simulink model "PV_MG_DroopMPPTVx_OneFarm"  (Simulink 8.5)
settings: Solver=ode3  StartTime=0.0  StopTime=inf  FixedStep=DT  RelTol=1e-3
PreLoadFcn:
  | DTCTinit;
PostLoadFcn:
  | Ts=50e-6;
InitFcn:
  | DTCTinit;
undefined symbols (not defined in the file): CT, DT
libraries: powerlib x25, simulink x6, powerlib_meascontrol x4, rtlab x2, simulink_extras x1, re_lib x1
settings Model: Creator=Nady  LastModifiedBy=ga63vey  PauseTimes=1.45  CovModelRefEnable=off
settings DataIOCC: SaveFormat=StructureWithTime  SignalLoggingSaveFormat=Dataset
settings OptimizationCC: ExpressionDepthLimit=128
settings DebuggingCC: UnderspecifiedInitializationDetection=Simplified  MergeDetectMultiDrivingBlocksExec=error  FcnCallInpInsideContextMsg=EnableAllAsError  StateNameClashWarn=none
settings HardwareCC: ProdBitPerPointer=64  ProdLargestAtomicFloat=Float  ProdIntDivRoundTo=Zero  ProdEndianess=LittleEndian  ProdHWDeviceType=Specified
settings GRTTargetCC: GeneratePreprocessorConditionals=Use local settings  CombineOutputUpdateFcns=on  GRTInterface=off

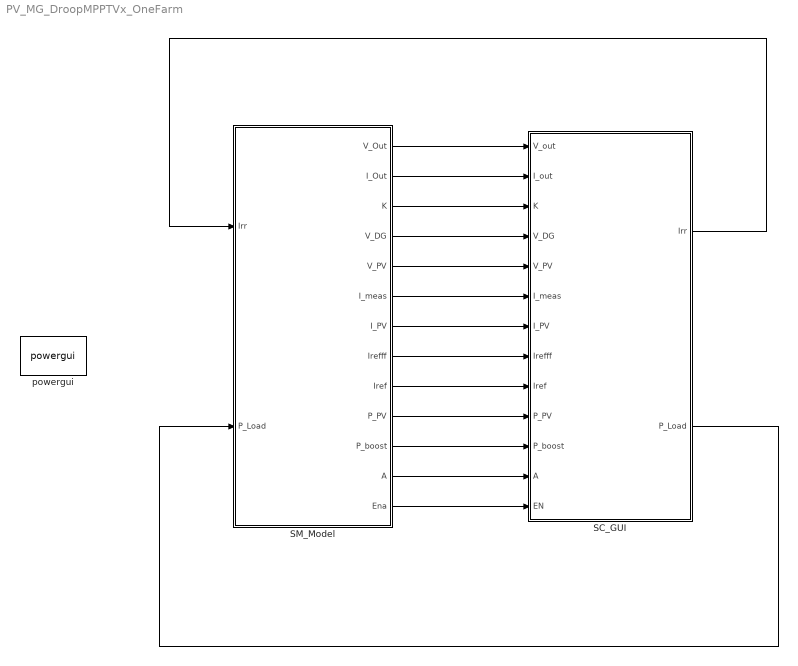
== system PV_MG_DroopMPPTVx_OneFarm ==
  SC_GUI : Subsystem
  SM_Model : Subsystem
  powergui : powerlib/powergui  Priority=1  SimulationMode=Discrete  SolverType=Tustin  SampleTime=DT  frequency=60  SPID=off  DisableSnubberDevices=off  DisableRonSwitches=off  DisableVfSwitches=off  SwTol=0  DisplayEquations=off  Interpol=off  methode=on  Ts=20  FunctionMessages=off  echomessages=off  HookPort=off  EnableUseOfTLC=off  x0status=blocks  frequencyindice=0  Pbase=100e6  ErrMax=1e-4  Iterations=50  UnitsV=kV  UnitsW=MW  buscounter=0  RestoreLinks=warning  ResistiveCurrentMeasurement=off  Frange=[0:2:500]  Ylog=off  Xlog=on  ShowGrid=off  save=off  variable=ZData  structure=0  ZoomFFT=off  StartTime=0.0  cycles=1  DisplayStyle=1  fundamental=60  FreqAxis=off  MaxFrequency=1000  frequencyindicesteady=1  RmsSteady=1  display=off
  wires:
  SC_GUI/1(Irr) -> SM_Model/1(Irr)
  SC_GUI/2(P_Load) -> SM_Model/2(P_Load)
  SM_Model/1(V_Out) -> SC_GUI/1(V_out)
  SM_Model/2(I_Out) -> SC_GUI/2(I_out)
  SM_Model/3(K) -> SC_GUI/3(K)
  SM_Model/4(V_DG) -> SC_GUI/4(V_DG)
  SM_Model/5(V_PV) -> SC_GUI/5(V_PV)
  SM_Model/6(I_meas) -> SC_GUI/6(I_meas)
  SM_Model/7(I_PV) -> SC_GUI/7(I_PV)
  SM_Model/8(Irefff) -> SC_GUI/8(Irefff)
  SM_Model/9(Iref) -> SC_GUI/9(Iref)
  SM_Model/10(P_PV) -> SC_GUI/10(P_PV)
  SM_Model/11(P_boost) -> SC_GUI/11(P_boost)
  SM_Model/12(A) -> SC_GUI/12(A)
  SM_Model/13(Ena) -> SC_GUI/13(EN)

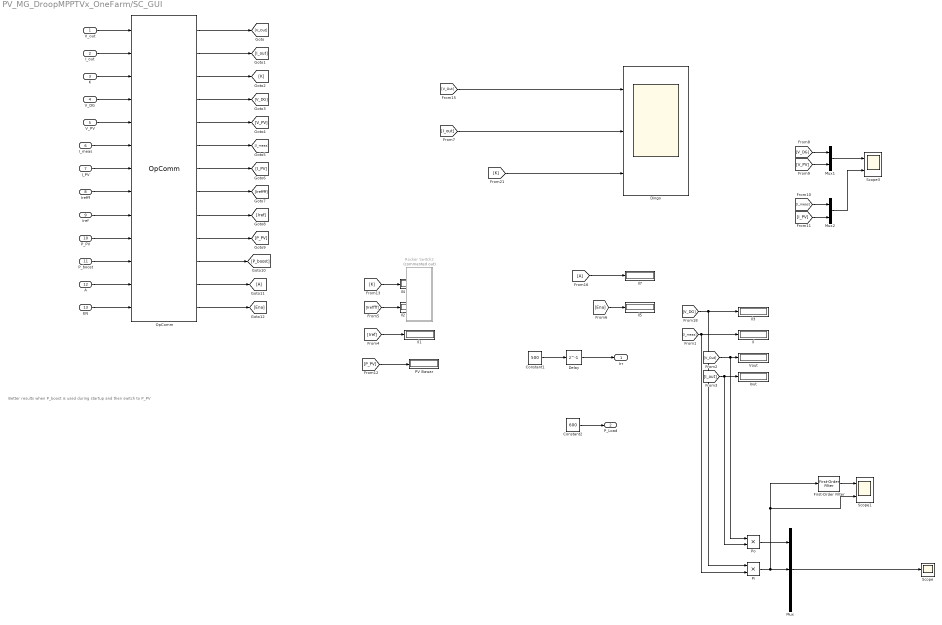
== system PV_MG_DroopMPPTVx_OneFarm/SC_GUI ==
  note: Better results when P_boost is used during startup and then switch to P_PV
  V_out : Inport
  I_out : Inport  Port=2
  K : Inport  Port=3
  V_DG : Inport  Port=4
  V_PV : Inport  Port=5
  I_meas : Inport  Port=6
  I_PV : Inport  Port=7
  Irefff : Inport  Port=8
  Iref : Inport  Port=9
  P_PV : Inport  Port=10
  P_boost : Inport  Port=11
  A : Inport  Port=12
  EN : Inport  Port=13
  Constant1 : Constant  Value=500  SampleTime=0
  Constant2 : Constant  Value=600  SampleTime=0
  Delay : Delay  DelayLength=1  InitialCondition=0
  Dingo : Scope  NumInputPorts=3
      settings: ShowLegends=on  TimeRange=3.8087  YMin=0~0~0  YMax=400~1.2~1.4  MaxDataPoints=10000
  First-Order Filter : powerlib_meascontrol/Filters/First-Order Filter  FilterType=Lowpass  Tc=1/400  Ts=DT  Initialize=off  Vac_Init=[0, 0, 60]  Vdc_Init=0  PlotResponse=off  FreqRange="[0,  200,  1]"
  Il{,1..5,7} (7 alike) : Display
  Iout : Display
  Mux : Mux  Inputs=3
  Mux1 : Mux  Inputs=2
  Mux2 : Mux  Inputs=2
  OpComm : rtlab/OpComm  nbport=13  groupe_acq=1  subsys_rate=0  st=0  Synchronization=on  Interpolation=on  Threshold=1.0  Missed_Data=off  Sim_Time=off  Samples=off  dynSigOut=off  from_console=0  warning_done=off  writeOpCommFile=off  Offset=off
  PV Bawar : Display
  Pi : Product
  Po : Product
  Rocker Switch2 : Subsystem  Commented=on  DialogController=hmiCreateDDGDialog  DialogControllerArgs=DataTag0  mask(MWDashboardBlock){webBlockId=5e99b1b3-df07-4cef-a3f6-0ddfeeb3b4e9, webBlockType=rockerswitch, ShowInLibBrowser=on, ShowInitialText=on, HMISrcModelName=[]}
      mask prompts: webBlockId "WebBlock Id"; webBlockType "WebBlock Type"; HMISrcModelName "Source Model"
      mask Help: helpview([docroot '/mapfiles/simulink.map'], 'hmi_rocker_switch')
      mask Display:
      | if strcmp(get_param(bdroot(gcb),'BlockDiagramType'), 'library')
      |     image([(matlabroot) '/toolbox/simulink/hmi/icons/RockerSwitch.png']);
      | end
  Scope : Scope
      settings: ShowLegends=on  YMin=-107.077  YMax=623.287  MaxDataPoints=10000
  Scope1 : Scope  NumInputPorts=2
      settings: YMin=-102.309~-5  YMax=495.80827~5
  Scope3 : Scope  NumInputPorts=2
      settings: YMin=-2.6975~-3.12322  YMax=24.27751~28.10897  SaveName=ScopeData3
  Vout : Display
  Irr : Outport
  P_Load : Outport  Port=2
  wires:
  [I_meas] -> Pi/2, Il/1
  [V_Out] -> Po/1, Vout/1
  [I_out] -> Po/2, Iout/1
  [V_DG] -> Il3/1, Pi/1
  Po/1 -> Mux/1
  Pi/1 -> First-Order Filter/1, Scope1/2, Mux/2
  [Iref] -> Il1/1
  [Ireffff] -> Il2/1
  [Ena] -> Il5/1
  First-Order Filter/1 -> Scope1/1
  Mux1/1 -> Scope3/1
  [V_DG] -> Mux1/1
  [V_PV] -> Mux1/2
  Mux2/1 -> Scope3/2
  [I_meas] -> Mux2/1
  [I_PV] -> Mux2/2
  [P_PV] -> PV Bawar/1
  [K] -> Il4/1
  Mux/1 -> Scope/1
  [K] -> Dingo/3
  [V_Out] -> Dingo/1
  [I_out] -> Dingo/2
  Constant1/1 -> Delay/1
  [A] -> Il7/1
  Delay/1 -> Irr/1
  V_out/1 -> OpComm/1
  I_out/1 -> OpComm/2
  K/1 -> OpComm/3
  V_DG/1 -> OpComm/4
  V_PV/1 -> OpComm/5
  I_meas/1 -> OpComm/6
  I_PV/1 -> OpComm/7
  Irefff/1 -> OpComm/8
  Iref/1 -> OpComm/9
  P_PV/1 -> OpComm/10
  P_boost/1 -> OpComm/11
  OpComm/1 -> [V_Out]
  OpComm/2 -> [I_out]
  OpComm/3 -> [K]
  OpComm/4 -> [V_DG]
  OpComm/5 -> [V_PV]
  OpComm/6 -> [I_meas]
  OpComm/7 -> [I_PV]
  OpComm/8 -> [Ireffff]
  OpComm/9 -> [Iref]
  OpComm/10 -> [P_PV]
  OpComm/11 -> [P_boost]
  OpComm/12 -> [A]
  OpComm/13 -> [Ena]
  A/1 -> OpComm/12
  EN/1 -> OpComm/13
  Constant2/1 -> P_Load/1

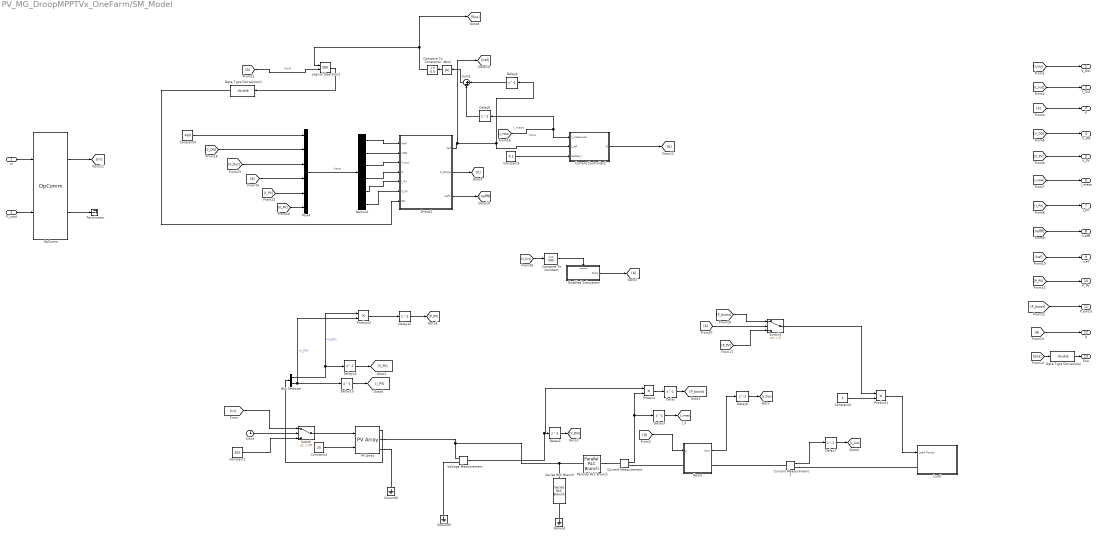
== system PV_MG_DroopMPPTVx_OneFarm/SM_Model ==
  note: here
  note: here
  note: here
  note: I_meas
  Irr : Inport
  P_Load : Inport  Port=2
  Abs2 : Abs
  Boost : Subsystem
  Bus Selector : BusSelector  OutputSignals=V_PV,I_PV
  Clock : Clock
  Compare To Constant : simulink/Logic and Bit Operations/Compare To Constant  relop=>=  const=395  OutDataTypeStr=boolean
  Compare To Constant2 : simulink/Logic and Bit Operations/Compare To Constant  relop=<=  const=0.5  OutDataTypeStr=boolean
  Constant1 : Constant  Value=400  SampleTime=0
  Constant2 : Constant  Value=25
  Constant3 : Constant  SampleTime=0
  Constant4 : Constant  Value=400  SampleTime=DT
  Constant5 : Constant  Value=0.1  SampleTime=CT
  Current Controller2 : Subsystem  TreatAsAtomicUnit=on
  Current Measurement : powerlib/Measurements/Current Measurement  PhasorSimulation=off  OutputType=Complex  PSBequivalent=0
  Current Measurement1 : powerlib/Measurements/Current Measurement  PhasorSimulation=off  OutputType=Complex  PSBequivalent=0
  Data Type Conversion : DataTypeConversion  OutDataTypeStr=double
  Data Type Conversion1 : DataTypeConversion  OutDataTypeStr=double
  Delay{,2..7,12..14} (10 alike) : Delay  DelayLength=1  InitialCondition=0
  Demux1 : Demux  Outputs=6
  Droop2 : Subsystem  TreatAsAtomicUnit=on
  Enabled Subsystem : Subsystem  TreatAsAtomicUnit=on
  Ground : powerlib/Elements/Ground  LConnTagsString=a
  Ground2 : powerlib/Elements/Ground  LConnTagsString=a
  Ground3 : powerlib/Elements/Ground  LConnTagsString=a
  Load : Subsystem
  Logical Operator2 : Logic  Operator=OR  AllPortsSameDT=off  OutDataTypeStr=boolean
  Mux4 : Mux  Inputs=6
  OpComm : rtlab/OpComm  nbport=2  groupe_acq=1  subsys_rate=0  st=0  Synchronization=on  Interpolation=on  Threshold=1.0  Missed_Data=off  Sim_Time=off  Samples=off  dynSigOut=off  from_console=1  warning_done=off  writeOpCommFile=off  Offset=off
  PV Array : re_lib/Solar/PV Array  Npar=5  Nser=1  PlotType=one module @ 25 deg.C & specified irradiances  S_vec="[ 1000  800 ]"  Temp_C_vec=[35]  ModuleName=Sun Earth Solar Power TDB125x125-36-P 80W  PlotWhenSelected=off  Pm=80.004  Ncell=36  Voc=21.9  Isc=5  Vm=17.7  Im=4.52  beta_Voc_pc=-0.32  alpha_Isc_pc=0.04  beta_Voc=-0.07008  alpha_Isc=0.002  IL=5.0238  I0=3.6974e-11  nI=0.92596  Rsh=70.2892  Rs=0.35567  BAL=on  Tc=1e-6  Tfilter=5e-5
  Parallel RLC Branch : powerlib/Elements/Parallel RLC Branch  LConnTagsString=a  RConnTagsString=__new0  BranchType=RL  Resistance=10  Inductance=0.0164  SetiL0=off  InitialCurrent=0  Capacitance=1e-6  Setx0=off  InitialVoltage=0  Measurements=None
  Product : Product
  Product1 : Product
  Product2 : Product
  Series RLC Branch : powerlib/Elements/Series RLC Branch  LConnTagsString=__new0  RConnTagsString=__new0  BranchType=C  Resistance=0.1  Inductance=1e-3  SetiL0=off  InitialCurrent=0  Capacitance=0.1  Setx0=off  InitialVoltage=0  Measurements=None
  Sum2 : Sum  Inputs=|+-
  Switch : Switch  Criteria=u2 > Threshold  Threshold=DT
  Switch1 : Switch  Criteria=u2 > Threshold
  Terminator : Terminator
  Voltage Measurement : powerlib/Measurements/Voltage Measurement  PhasorSimulation=off  OutputType=Complex  PSBequivalent=0
  V_Out : Outport
  I_Out : Outport  Port=2
  K : Outport  Port=3
  V_DG : Outport  Port=4
  V_PV : Outport  Port=5
  I_meas : Outport  Port=6
  I_PV : Outport  Port=7
  Irefff : Outport  Port=8
  Iref : Outport  Port=9
  P_PV : Outport  Port=10
  P_boost : Outport  Port=11
  A : Outport  Port=12
  Ena : Outport  Port=13
  wires:
  Droop2/1(Iref) -> [Iref], Delay4/1, Current Controller2/2(I_ref)
  Constant5/1 -> Current Controller2/3(delata_I)
  Droop2/2(K_droop) -> [K]
  Droop2/3(Iref1) -> [Ireffff]
  Sum2/1 -> Abs2/1
  Abs2/1 -> Compare To Constant2/1
  Delay4/1 -> Sum2/1
  Delay5/1 -> Sum2/2
  Constant4/1 -> Mux4/1
  [V_DG] -> Mux4/2
  [V_Out] -> Mux4/3
  Current Controller2/1(G) -> [G]
  Compare To Constant2/1 -> [Ena], Logical Operator2/1
  Logical Operator2/1 -> Data Type Conversion1/1
  Data Type Conversion1/1 -> Droop2/7(EN)
  Demux1/1 -> Droop2/1(Vref)
  Demux1/2 -> Droop2/2(vDG)
  Demux1/3 -> Droop2/3(V_out)
  Demux1/4 -> Droop2/4(A)
  Demux1/5 -> Droop2/5(I_PV)
  Demux1/6 -> Droop2/6(V_PV)
  [A] -> Mux4/4
  [I_PV] -> Mux4/5
  [V_PV] -> Mux4/6
  Boost/1(Vout) -> Delay6/1
  Voltage Measurement/1 -> Delay2/1, Product/1
  Current Measurement/1 -> Product/2, Delay3/1
  Product1/1 -> Load/1(Load Power)
  Current Measurement1/1 -> Delay7/1
  Product/1 -> Delay/1
  Delay/1 -> [P_boost]
  Delay2/1 -> [V_DG]
  Delay3/1 -> [I_meas]
  Delay6/1 -> [V_Out]
  Delay7/1 -> [I_out]
  Constant2/1 -> PV Array/2
  Bus Selector/1 -> Delay14/1, Product2/1  "<V_PV>"
  Bus Selector/2 -> Delay13/1, Product2/2  "<I_PV>"
  PV Array/1 -> Bus Selector/1
  Product2/1 -> Delay12/1
  Delay12/1 -> [P_PV]
  [G] -> Boost/1(g)
  Delay13/1 -> [I_PV]
  Delay14/1 -> [V_PV]
  [Irr] -> Switch/1
  Switch/1 -> PV Array/1
  Clock/1 -> Switch/2
  Enabled Subsystem/1(Out1) -> [A]
  [V_Out] -> Compare To Constant/1
  Compare To Constant/1 -> Enabled Subsystem/Enable
  Irr/1 -> OpComm/1
  P_Load/1 -> OpComm/2
  OpComm/1 -> [Irr]
  OpComm/2 -> Terminator/1
  [V_Out] -> V_Out/1
  [I_out] -> I_Out/1
  [K] -> K/1
  [V_DG] -> V_DG/1
  [V_PV] -> V_PV/1
  [I_meas] -> I_meas/1
  [I_PV] -> I_PV/1
  [Ireffff] -> Irefff/1
  [Iref] -> Iref/1
  [P_PV] -> P_PV/1
  [A] -> A/1
  [P_boost] -> P_boost/1
  [Ena] -> Data Type Conversion/1
  Data Type Conversion/1 -> Ena/1
  Constant1/1 -> Switch/3
  Mux4/1 -> Demux1/1
  [A] -> Logical Operator2/2
  [I_meas] -> Current Controller2/1(I_measured), Delay5/1
  [P_boost] -> Switch1/1
  [P_PV] -> Switch1/3
  Switch1/1 -> Product1/1
  Constant3/1 -> Product1/2
  [A] -> Switch1/2
  connections:
  Series RLC Branch/LConn1 -- Parallel RLC Branch/LConn1 -- Voltage Measurement/LConn1 -- PV Array/RConn1
  Parallel RLC Branch/RConn1 -- Current Measurement/LConn1
  Ground/LConn1 -- Series RLC Branch/RConn1
  Current Measurement1/RConn1 -- Load/LConn1
  Boost/RConn1 -- Current Measurement1/LConn1
  Current Measurement/RConn1 -- Boost/LConn1
  Voltage Measurement/LConn2 -- Ground3/LConn1
  PV Array/RConn2 -- Ground2/LConn1

== system PV_MG_DroopMPPTVx_OneFarm/SC_GUI/Rocker Switch2 ==

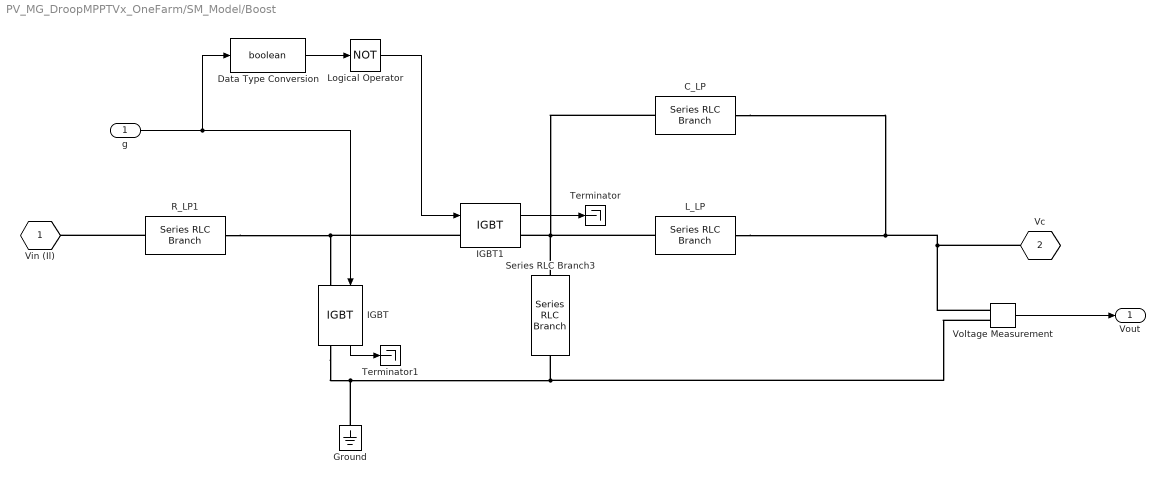
== system PV_MG_DroopMPPTVx_OneFarm/SM_Model/Boost ==
  g : Inport
  C_LP : powerlib/Elements/Series RLC Branch  LConnTagsString=__new0  RConnTagsString=__new0  BranchType=R  Resistance=1  Inductance=1e-3  SetiL0=off  InitialCurrent=0  Capacitance=0.004  Setx0=off  InitialVoltage=0  Measurements=None
  Data Type Conversion : DataTypeConversion  OutDataTypeStr=boolean
  Ground : powerlib/Elements/Ground  LConnTagsString=a
  IGBT : powerlib/Power Electronics/IGBT  Ron=0.001  Lon=0  Vf=1  Tf=1e-6  Tt=2e-6  IC=0  Rs=1e5  Cs=inf  Measurements=on
  IGBT1 : powerlib/Power Electronics/IGBT  Ron=0.001  Lon=0  Vf=1  Tf=1e-6  Tt=2e-6  IC=0  Rs=1e5  Cs=inf  Measurements=on
  L_LP : powerlib/Elements/Series RLC Branch  LConnTagsString=__new0  RConnTagsString=__new0  BranchType=L  Resistance=0.01  Inductance=0.0164  SetiL0=off  InitialCurrent=0  Capacitance=6e-2  Setx0=off  InitialVoltage=0  Measurements=None
  Logical Operator : Logic  Operator=NOT  AllPortsSameDT=off  OutDataTypeStr=boolean
  R_LP1 : powerlib/Elements/Series RLC Branch  LConnTagsString=__new0  RConnTagsString=__new0  BranchType=L  Resistance=0.01  Inductance=7e-3  SetiL0=off  InitialCurrent=0  Capacitance=6e-2  Setx0=off  InitialVoltage=0  Measurements=None
  Series RLC Branch3 : powerlib/Elements/Series RLC Branch  LConnTagsString=__new0  RConnTagsString=__new0  BranchType=C  Resistance=0.005  Inductance=1e-3  SetiL0=off  InitialCurrent=0  Capacitance=1e-2  Setx0=off  InitialVoltage=0  Measurements=None
  Terminator : Terminator
  Terminator1 : Terminator
  Voltage Measurement : powerlib/Measurements/Voltage Measurement  PhasorSimulation=off  OutputType=Complex  PSBequivalent=0
  Vin (Il) : PMIOPort  Tag=PMCPort  Port=1  Side=Left
  Vc : PMIOPort  Tag=PMCPort  Port=2  Side=Right
  Vout : Outport
  wires:
  Voltage Measurement/1 -> Vout/1
  g/1 -> Data Type Conversion/1, IGBT/1
  Data Type Conversion/1 -> Logical Operator/1
  Logical Operator/1 -> IGBT1/1
  IGBT1/1 -> Terminator/1
  IGBT/1 -> Terminator1/1
  connections:
  IGBT/RConn1 -- Ground/LConn1 -- Voltage Measurement/LConn2 -- Series RLC Branch3/RConn1
  IGBT1/LConn1 -- R_LP1/LConn1 -- IGBT/LConn1
  R_LP1/RConn1 -- Vin (Il)/RConn1
  Vc/RConn1 -- L_LP/LConn1 -- C_LP/LConn1 -- Voltage Measurement/LConn1
  C_LP/RConn1 -- L_LP/RConn1 -- Series RLC Branch3/LConn1 -- IGBT1/RConn1

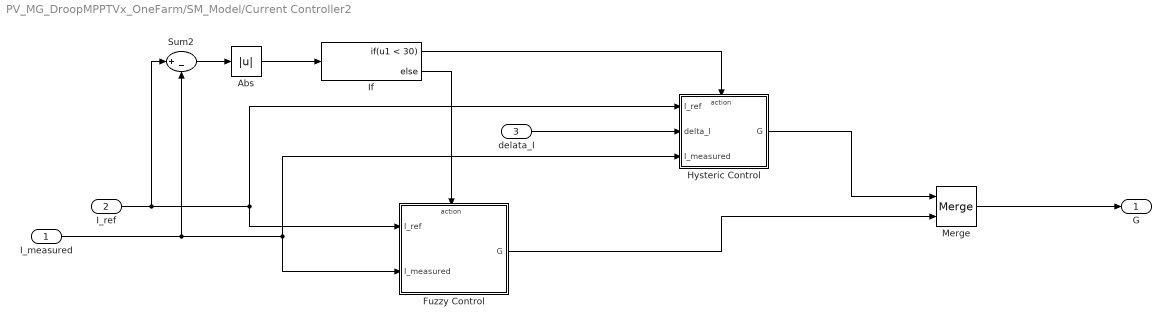
== system PV_MG_DroopMPPTVx_OneFarm/SM_Model/Current Controller2 ==
  I_measured : Inport  SampleTime=CT
  I_ref : Inport  Port=2  SampleTime=CT
  delata_I : Inport  Port=3
  Abs : Abs
  Fuzzy Control : Subsystem  TreatAsAtomicUnit=on
  Hysteric Control : Subsystem  TreatAsAtomicUnit=on
  If : If  IfExpression=u1 < 30
  Merge : Merge
  Sum2 : Sum  Inputs=|+-
  G : Outport
  wires:
  Merge/1 -> G/1
  Abs/1 -> If/1
  Sum2/1 -> Abs/1
  Hysteric Control/1(G) -> Merge/1
  delata_I/1 -> Hysteric Control/2(delta_I)
  Fuzzy Control/1(G) -> Merge/2
  I_measured/1 -> Sum2/2, Fuzzy Control/2(I_measured), Hysteric Control/3(I_measured)
  I_ref/1 -> Fuzzy Control/1(I_ref), Hysteric Control/1(I_ref), Sum2/1
  If/2 -> Fuzzy Control/Action
  If/1 -> Hysteric Control/Action

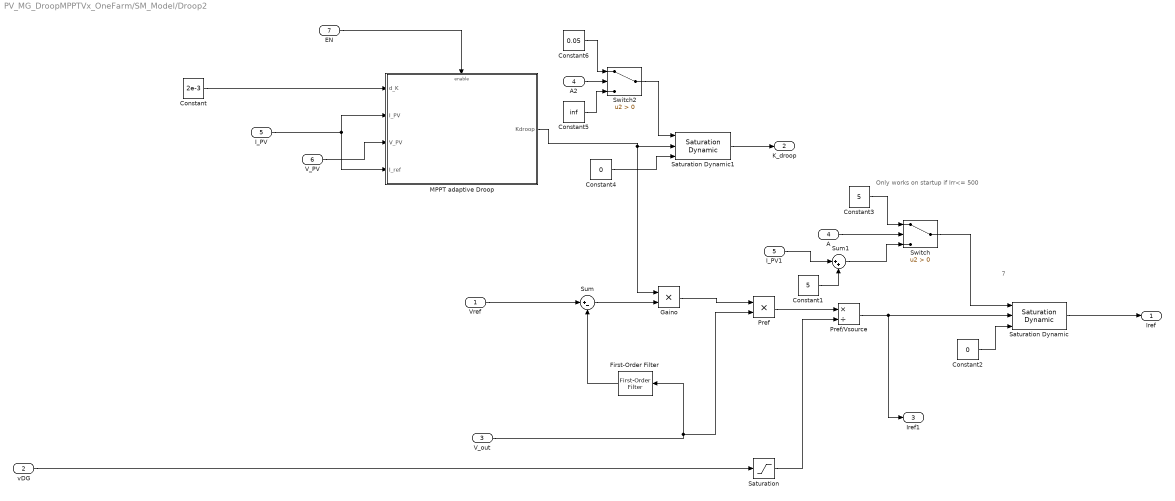
== system PV_MG_DroopMPPTVx_OneFarm/SM_Model/Droop2 ==
  note: Only works on startup if Irr<= 500
  note: 7
  Vref : Inport  SampleTime=CT
  vDG : Inport  Port=2  SampleTime=CT
  V_out : Inport  Port=3  SampleTime=CT
  A : Inport  Port=4  SampleTime=CT
  I_PV : Inport  Port=5  SampleTime=CT
  V_PV : Inport  Port=6
  EN : Inport  Port=7
  A2 : InportShadow  Port=4  SampleTime=CT
  Constant : Constant  Value=2e-3  SampleTime=CT
  Constant1 : Constant  Value=5  SampleTime=CT
  Constant2 : Constant  Value=0  SampleTime=CT
  Constant3 : Constant  Value=5  SampleTime=CT
  Constant4 : Constant  Value=0  SampleTime=CT
  Constant5 : Constant  Value=inf  SampleTime=CT
  Constant6 : Constant  Value=0.05  SampleTime=CT
  First-Order Filter : powerlib_meascontrol/Filters/First-Order Filter  FilterType=Lowpass  Tc=1/8000  Ts=CT  Initialize=off  Vac_Init=[0, 0, 60]  Vdc_Init=0  PlotResponse=off  FreqRange="[0,  5000,  1]"
  Gaino : Product
  I_PV1 : InportShadow  Port=5  SampleTime=CT
  MPPT adaptive Droop : Subsystem  TreatAsAtomicUnit=on
  Pref : Product
  Pref/Vsource : Product  Inputs=*/
  Saturation : Saturate  UpperLimit=inf  LowerLimit=1
  Saturation Dynamic : simulink/Discontinuities/Saturation Dynamic  OutMin=[]  OutMax=[]  OutDataTypeStr=Inherit: Same as second input  OutDataType=fixdt(1, 16)  OutScaling=2^-10  DoSatur=off
  Saturation Dynamic1 : simulink/Discontinuities/Saturation Dynamic  OutMin=[]  OutMax=[]  OutDataTypeStr=Inherit: Same as second input  OutDataType=fixdt(1, 16)  OutScaling=2^-10  DoSatur=off
  Sum : Sum  Inputs=|+-
  Sum1 : Sum  Inputs=|++
  Switch : Switch  Criteria=u2 > Threshold
  Switch2 : Switch  Criteria=u2 > Threshold
  Iref : Outport  SampleTime=CT
  K_droop : Outport  Port=2
  Iref1 : Outport  Port=3
  wires:
  MPPT adaptive Droop/1(Kdroop) -> Saturation Dynamic1/2, Gaino/1
  I_PV/1 -> MPPT adaptive Droop/2(I_PV), MPPT adaptive Droop/4(I_ref)
  V_PV/1 -> MPPT adaptive Droop/3(V_PV)
  EN/1 -> MPPT adaptive Droop/Enable
  vDG/1 -> Saturation/1
  Constant/1 -> MPPT adaptive Droop/1(d_K)
  A/1 -> Switch/2
  Sum1/1 -> Switch/3
  Switch/1 -> Saturation Dynamic/1
  Constant2/1 -> Saturation Dynamic/3
  Vref/1 -> Sum/1
  V_out/1 -> First-Order Filter/1, Pref/2
  Pref/Vsource/1 -> Iref1/1, Saturation Dynamic/2
  Gaino/1 -> Pref/1
  Saturation/1 -> Pref/Vsource/2
  Pref/1 -> Pref/Vsource/1
  First-Order Filter/1 -> Sum/2
  Sum/1 -> Gaino/2
  Saturation Dynamic1/1 -> K_droop/1
  Switch2/1 -> Saturation Dynamic1/1
  A2/1 -> Switch2/2
  Constant4/1 -> Saturation Dynamic1/3
  Constant5/1 -> Switch2/3
  Constant6/1 -> Switch2/1
  I_PV1/1 -> Sum1/1
  Constant1/1 -> Sum1/2
  Saturation Dynamic/1 -> Iref/1
  Constant3/1 -> Switch/1

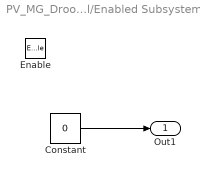
== system PV_MG_DroopMPPTVx_OneFarm/SM_Model/Enabled Subsystem ==
  Enable : EnablePort
  Constant : Constant  Value=0
  Out1 : Outport  InitialOutput=1
  wires:
  Constant/1 -> Out1/1

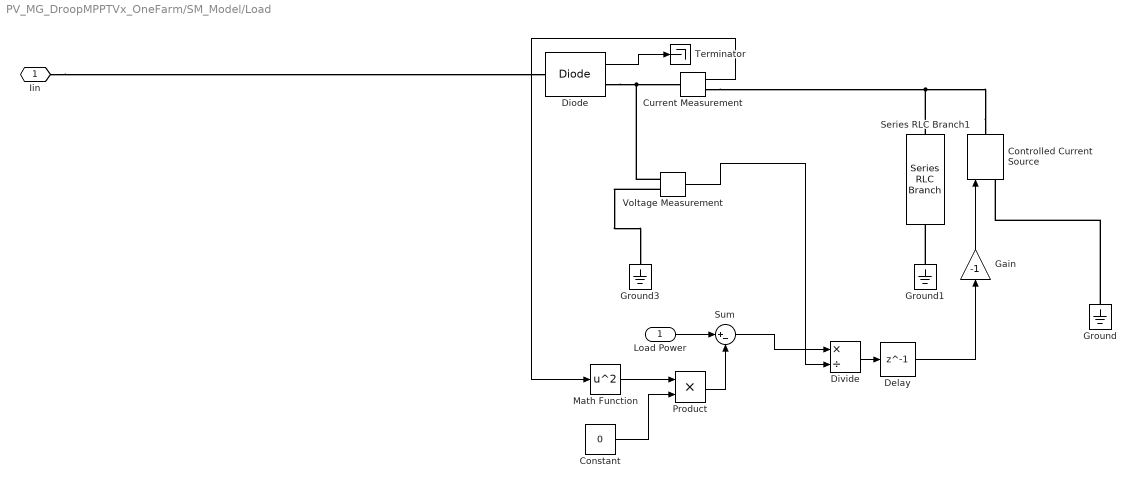
== system PV_MG_DroopMPPTVx_OneFarm/SM_Model/Load ==
  Load Power : Inport
  Constant : Constant  Value=0
  Controlled Current Source : powerlib/Electrical Sources/Controlled Current Source  Initialize=on  Source_Type=AC  Amplitude=0  Phase=0  Frequency=0  Measurements=None
  Current Measurement : powerlib/Measurements/Current Measurement  PhasorSimulation=off  OutputType=Complex  PSBequivalent=0
  Delay : Delay  DelayLength=1  InitialCondition=0
  Diode : powerlib/Power Electronics/Diode  Ron=0.001  Lon=0  Vf=0.8  IC=0  UseSnubber=off  Rs=500  Cs=250e-9  Measurements=on
  Divide : Product  Inputs=*/
  Gain : Gain  Gain=-1
  Ground : powerlib/Elements/Ground  LConnTagsString=a
  Ground1 : powerlib/Elements/Ground  LConnTagsString=a
  Ground3 : powerlib/Elements/Ground  LConnTagsString=a
  Math Function : Math  Operator=square  SaturateOnIntegerOverflow=on
  Product : Product
  Series RLC Branch1 : powerlib/Elements/Series RLC Branch  LConnTagsString=__new0  RConnTagsString=__new0  BranchType=C  Resistance=1  Inductance=1e-3  SetiL0=off  InitialCurrent=0  Capacitance=1e-3  Setx0=off  InitialVoltage=0  Measurements=None
  Sum : Sum  Inputs=|+-
  Terminator : Terminator
  Voltage Measurement : powerlib/Measurements/Voltage Measurement  PhasorSimulation=off  OutputType=Complex  PSBequivalent=0
  Iin : PMIOPort  Port=1  Side=Left
  wires:
  Gain/1 -> Controlled Current Source/1
  Divide/1 -> Delay/1
  Delay/1 -> Gain/1
  Math Function/1 -> Product/1
  Constant/1 -> Product/2
  Load Power/1 -> Sum/1
  Product/1 -> Sum/2
  Sum/1 -> Divide/1
  Current Measurement/1 -> Math Function/1
  Voltage Measurement/1 -> Divide/2
  Diode/1 -> Terminator/1
  connections:
  Voltage Measurement/LConn1 -- Diode/RConn1 -- Current Measurement/LConn1
  Voltage Measurement/LConn2 -- Ground3/LConn1
  Ground/LConn1 -- Controlled Current Source/LConn1
  Controlled Current Source/RConn1 -- Current Measurement/RConn1 -- Series RLC Branch1/LConn1
  Ground1/LConn1 -- Series RLC Branch1/RConn1
  Iin/RConn1 -- Diode/LConn1

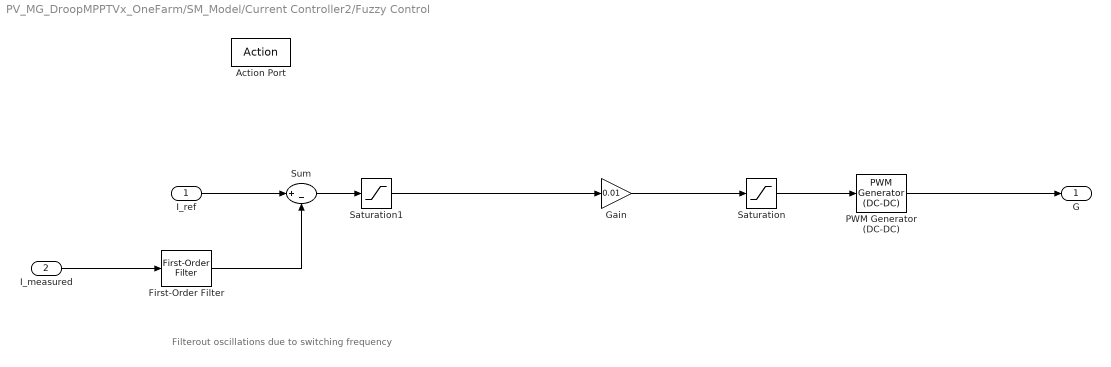
== system PV_MG_DroopMPPTVx_OneFarm/SM_Model/Current Controller2/Fuzzy Control ==
  note: Filterout oscillations due to switching frequency
  I_ref : Inport
  I_measured : Inport  Port=2
  Action Port : ActionPort  ActionType=else
  First-Order Filter : powerlib_meascontrol/Filters/First-Order Filter  FilterType=Lowpass  Tc=1/8000  Ts=CT  Initialize=off  Vac_Init=[0, 0, 60]  Vdc_Init=0  PlotResponse=off  FreqRange="[0,  5000,  1]"
  Gain : Gain  Gain=0.01
  PWM Generator (DC-DC) : powerlib_meascontrol/Pulse & Signal Generators/PWM Generator (DC-DC)  Fsw=10000  Ts=CT
  Saturation : Saturate  UpperLimit=0.8  LowerLimit=0
  Saturation1 : Saturate  UpperLimit=100  LowerLimit=-100
  Sum : Sum  Inputs=|+-
  G : Outport
  wires:
  First-Order Filter/1 -> Sum/2
  I_measured/1 -> First-Order Filter/1
  Saturation1/1 -> Gain/1
  Sum/1 -> Saturation1/1
  PWM Generator (DC-DC)/1 -> G/1
  Saturation/1 -> PWM Generator (DC-DC)/1
  I_ref/1 -> Sum/1
  Gain/1 -> Saturation/1

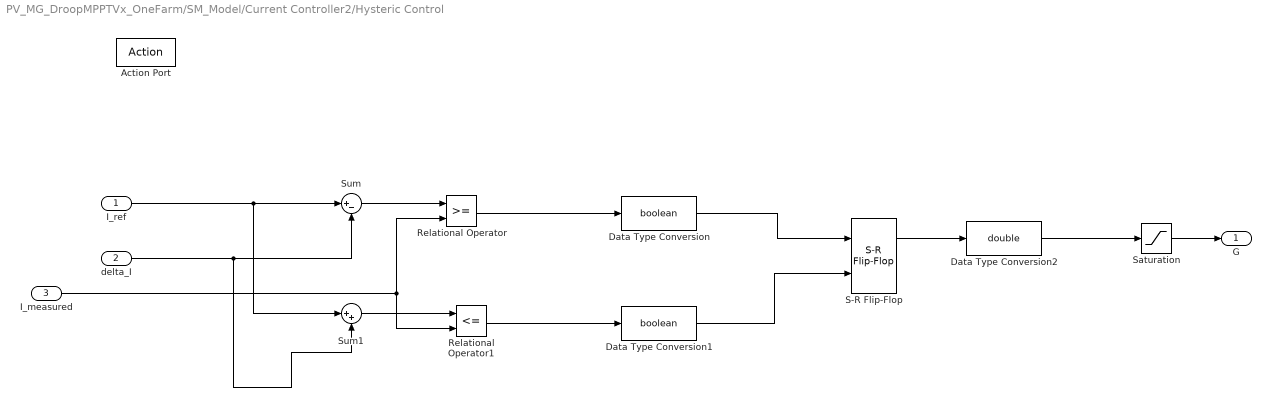
== system PV_MG_DroopMPPTVx_OneFarm/SM_Model/Current Controller2/Hysteric Control ==
  I_ref : Inport
  delta_I : Inport  Port=2
  I_measured : Inport  Port=3
  Action Port : ActionPort  ActionType=then
  Data Type Conversion : DataTypeConversion  OutDataTypeStr=boolean
  Data Type Conversion1 : DataTypeConversion  OutDataTypeStr=boolean
  Data Type Conversion2 : DataTypeConversion  OutDataTypeStr=double
  Relational Operator : RelationalOperator  OutDataTypeStr=boolean  ZeroCross=off
  Relational Operator1 : RelationalOperator  Operator=<=  OutDataTypeStr=boolean  ZeroCross=off
  S-R Flip-Flop : simulink_extras/Flip Flops/S-R Flip-Flop  initial_condition=0
  Saturation : Saturate  UpperLimit=1  LowerLimit=0
  Sum : Sum  Inputs=|+-
  Sum1 : Sum  Inputs=|++
  G : Outport
  wires:
  S-R Flip-Flop/1 -> Data Type Conversion2/1
  Saturation/1 -> G/1
  Data Type Conversion2/1 -> Saturation/1
  I_measured/1 -> Relational Operator1/2, Relational Operator/2
  Sum1/1 -> Relational Operator1/1
  Relational Operator1/1 -> Data Type Conversion1/1
  Relational Operator/1 -> Data Type Conversion/1
  Sum/1 -> Relational Operator/1
  Data Type Conversion1/1 -> S-R Flip-Flop/2
  Data Type Conversion/1 -> S-R Flip-Flop/1
  delta_I/1 -> Sum1/2, Sum/2
  I_ref/1 -> Sum/1, Sum1/1

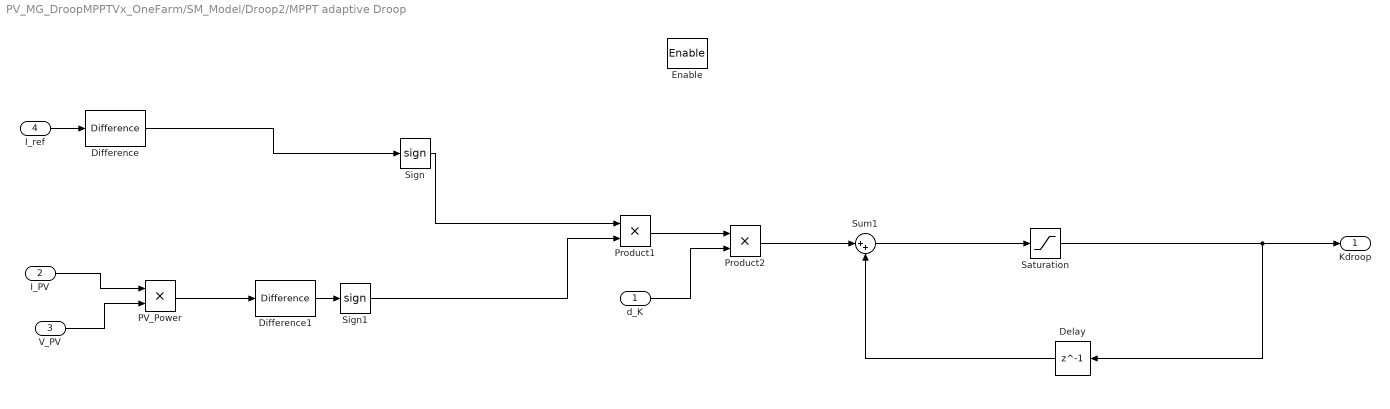
== system PV_MG_DroopMPPTVx_OneFarm/SM_Model/Droop2/MPPT adaptive Droop ==
  d_K : Inport  SampleTime=CT
  I_PV : Inport  Port=2  SampleTime=CT
  V_PV : Inport  Port=3  SampleTime=CT
  I_ref : Inport  Port=4  SampleTime=CT
  Enable : EnablePort
  Delay : Delay  DelayLength=1  InitialCondition=0  SampleTime=CT
  Difference : simulink/Discrete/Difference  ICPrevInput=0.0  InputProcessing=Inherited  OutMin=[]  OutMax=[]  OutDataType=fixdt(1, 16)  OutScaling=2^-10  DoSatur=off
  Difference1 : simulink/Discrete/Difference  ICPrevInput=0.0  InputProcessing=Inherited  OutMin=[]  OutMax=[]  OutDataType=fixdt(1, 16)  OutScaling=2^-10  DoSatur=off
  PV_Power : Product
  Product1 : Product
  Product2 : Product
  Saturation : Saturate  UpperLimit=4  LowerLimit=0
  Sign : Signum
  Sign1 : Signum
  Sum1 : Sum  Inputs=|++
  Kdroop : Outport  SampleTime=CT  InitialOutput=0.01
  wires:
  I_ref/1 -> Difference/1
  V_PV/1 -> PV_Power/2
  I_PV/1 -> PV_Power/1
  Difference/1 -> Sign/1
  Sum1/1 -> Saturation/1
  Delay/1 -> Sum1/2
  Product2/1 -> Sum1/1
  d_K/1 -> Product2/2
  Product1/1 -> Product2/1
  Sign1/1 -> Product1/2
  Difference1/1 -> Sign1/1
  PV_Power/1 -> Difference1/1
  Saturation/1 -> Delay/1, Kdroop/1
  Sign/1 -> Product1/1
